simulink model "GazeboDifferentialDriveControl"  (R2023b)
settings: Solver=VariableStepAuto  StartTime=0.0  StopTime=15  RelTol=1e-3
StopFcn:
  | robotPoses = out.yout{1}.Values.Data;
  | 
  | figure;
  | plot(waypoints(:,1), waypoints(:,2), 'k-x');
  | hold all
  | plot(robotPoses(:,1), robotPoses(:,2));
  | title('XY Waypoint Tracking');
undefined symbols (not defined in the file): duration, effort, index, joint_name, left_wheel_hinge, model_name, pioneer2dx, right_wheel_hinge, waypoints
libraries: robotgazebolib x10, robotalgslib x1, robotcorelib x1
settings Model: PacingRate=0.011000  Creator=The MathWorks, Inc.  LastModifiedBy=basit
settings SolverCC: AlgebraicLoopSolver=TrustRegion
settings DebuggingCC: UnconnectedInputMsg=warning  UnconnectedOutputMsg=warning  UnconnectedLineMsg=warning  SymbolicDimsDataTypeCodeGenerationDiagnostic=none
settings ModelReferenceCC: EnableRefExpFcnMdlSchedulingChecks=on

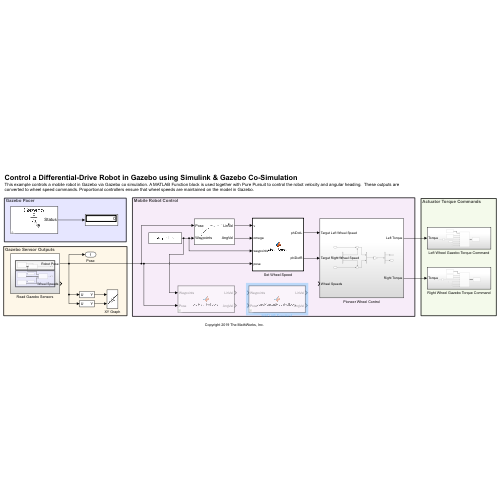
[thumbnail: Simulink's stored preview of the top-level diagram]
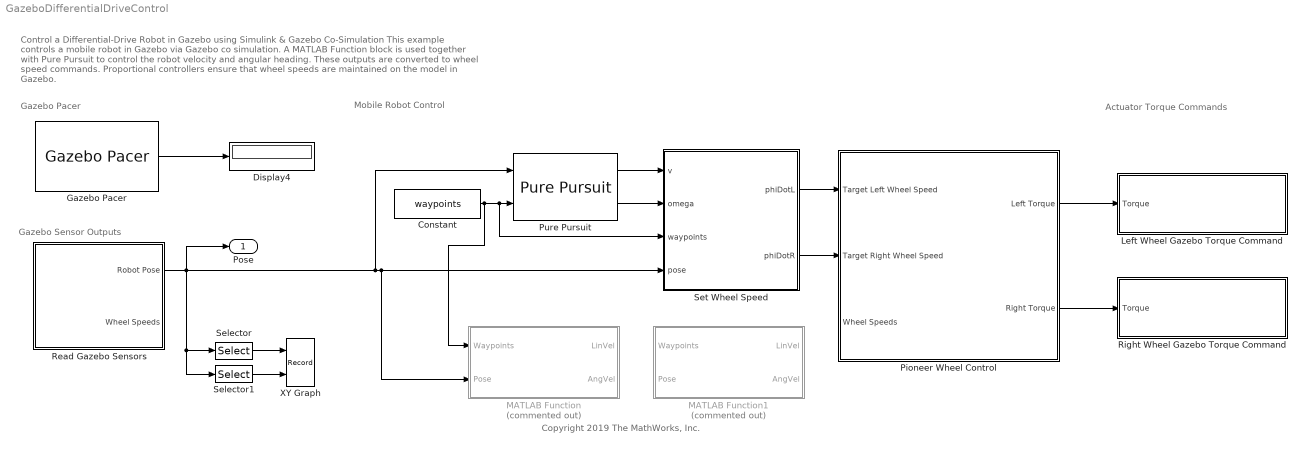
== system GazeboDifferentialDriveControl ==
  note: Gazebo Pacer
  note: Actuator Torque Commands
  note: Control a Differential-Drive Robot in Gazebo using Simulink & Gazebo Co-Simulation
      | This example controls a mobile robot in Gazebo via Gazebo co simulation. A MATLAB Function block is used together with Pure Pursuit to control the robot velocity and angular heading. These outputs are converted to wheel speed commands. Proportional controllers ensure that wheel speeds are maintained on the model in Gazebo.
  note: Copyright 2019 The MathWorks, Inc.
  note: Gazebo Sensor Outputs
  note: Mobile Robot Control
  Constant : Constant  Value=waypoints
  Display4 : Display
  Gazebo Pacer : robotgazebolib/Gazebo Pacer  ResetBehavior=Reset Gazebo simulation time and scene  SampleTime=0.01
  Left Wheel Gazebo Torque Command : Subsystem
  MATLAB Function : MATLAB Function  Commented=on  TreatAsAtomicUnit=on
  MATLAB Function1 : MATLAB Function  Commented=on  TreatAsAtomicUnit=on
  Pioneer Wheel Control : Subsystem
  Pure Pursuit : robotalgslib/Pure Pursuit  DesiredLinearVelocity=1  MaxAngularVelocity=1.0  LookaheadDistance=1.0  TargetDirPort=off  SimulateUsing=Code generation
  Read Gazebo Sensors : Subsystem
  Right Wheel Gazebo Torque Command : Subsystem
  Selector : Selector  InputPortWidth=3  IndexOptions=Index vector (dialog)  Indices=[1]  OutputSizes=1
  Selector1 : Selector  InputPortWidth=3  IndexOptions=Index vector (dialog)  Indices=[2]  OutputSizes=1
  Set Wheel Speed : MATLAB Function  TreatAsAtomicUnit=on
  XY Graph : Record  FileSettingsInternal="{\"entries\":[{\"content\":{\"excelSettings\":{\"content\":{},\"type\":\"Streamout.ExcelSettings\"}},\"type\":\"Streamout.FileSettingStorage\",\"uuid\":\"\"}],\"packageUris\":[\"http:\\/\\/schema.mathworks.com\\/mf0\\/streamout_blocks\\/R2020a\"],\"version\":\"1.0\"}"  Layout=[1 1]  SignalsInternal="{\"entries\":[{\"content\":{\"signals\":[{\"content\":{\"blockPath\":[],\"dimensions\":[1],\"domain\":\"\",\"lineColor\":\"#a2142f\",\"port\":1,\"signalID\":8,\"signalName\":\"XY Graph:1\"},\"type\":\"RecordBlkView.Signal\",\"uuid\":\"\"},{\"content\":{\"blockPath\":[],\"dimensions\":[1],\"domain\":\"\",\"lineColor\":\"#139fff\",\"plots\":[1],\"port\":2,\"signalID\":11,\"signalName\":\"XY Graph:2\"},\"type\":\"RecordBlkView.Signal\",\"uuid\":\"\"}]},\"type\":\"RecordBlkView.InputSignals\",\"uuid\":\"\"}],\"packageUris\":[\"http:\\/\\/schema.mathworks.com\\/mf0\\/streamout_blocks\\/R2020a\"],\"version\":\"1.0\"}"  VisualizationBindings="{\"xyplotplugin\":{\"info\":[{\"series\":[{\"bindingParametersList\":[{\"parameter\":\"Y-Axis\",\"signalID\":11,\"signalName\":\"XY Graph:2\"}],\"seriesID\":42836}],\"subplotID\":1}]}}"  CompatibilityTag=XY  st=-1
  Pose : Outport
  wires:
  Set Wheel Speed/1(phiDotL) -> Pioneer Wheel Control/1(Target Left Wheel Speed)
  Gazebo Pacer/1 -> Display4/1
  Constant/1 -> MATLAB Function/1(Waypoints), Set Wheel Speed/3(waypoints), Pure Pursuit/2
  Read Gazebo Sensors/1(Robot Pose) -> MATLAB Function/2(Pose), Set Wheel Speed/4(pose), Pure Pursuit/1, Pose/1, Selector/1, Selector1/1
  Pioneer Wheel Control/1(Left Torque) -> Left Wheel Gazebo Torque Command/1(Torque)
  Pioneer Wheel Control/2(Right Torque) -> Right Wheel Gazebo Torque Command/1(Torque)
  Selector/1 -> XY Graph/1
  Selector1/1 -> XY Graph/2
  Pure Pursuit/1 -> Set Wheel Speed/1(v)
  Pure Pursuit/2 -> Set Wheel Speed/2(omega)
  Set Wheel Speed/2(phiDotR) -> Pioneer Wheel Control/2(Target Right Wheel Speed)

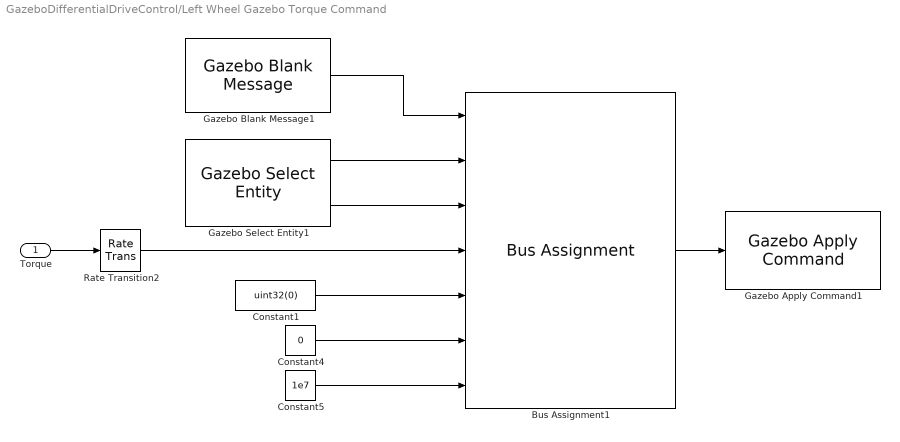
== system GazeboDifferentialDriveControl/Left Wheel Gazebo Torque Command ==
  Torque : Inport
  Bus Assignment1 : BusAssignment  AssignedSignals=model_name,joint_name,effort,index,duration.seconds,duration.nano_seconds
  Constant1 : Constant  Value=uint32(0)
  Constant4 : Constant  Value=0
  Constant5 : Constant  Value=1e7
  Gazebo Apply Command1 : robotgazebolib/Gazebo Apply Command  cmdType=ApplyJointTorque  sampleTime=0.01
  Gazebo Blank Message1 : robotgazebolib/Gazebo Blank Message  msgType=ApplyJointTorque  sampleTime=0.01  busName='Gazebo_SL_Bus_gazebo_msgs_ApplyJointTorque'
  Gazebo Select Entity1 : robotgazebolib/Gazebo Select Entity  modelElemName=pioneer2dx/left_wheel_hinge  outputArraySize=128  OutputLabel=Joint  SelectType=Joint
  Rate Transition2 : RateTransition
  wires:
  Bus Assignment1/1 -> Gazebo Apply Command1/1
  Constant5/1 -> Bus Assignment1/7
  Gazebo Blank Message1/1 -> Bus Assignment1/1
  Gazebo Select Entity1/2 -> Bus Assignment1/3
  Gazebo Select Entity1/1 -> Bus Assignment1/2
  Torque/1 -> Rate Transition2/1
  Constant4/1 -> Bus Assignment1/6
  Rate Transition2/1 -> Bus Assignment1/4
  Constant1/1 -> Bus Assignment1/5

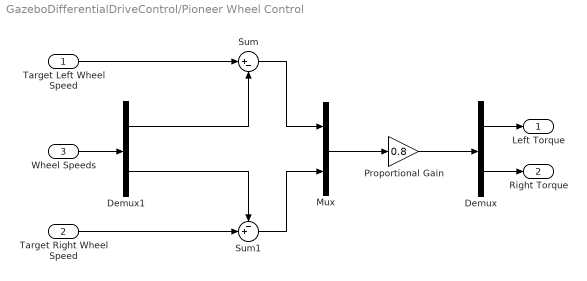
== system GazeboDifferentialDriveControl/Pioneer Wheel Control ==
  Target Left Wheel Speed : Inport
  Target Right Wheel Speed : Inport  Port=2
  Wheel Speeds : Inport  Port=3
  Demux : Demux  Outputs=2
  Demux1 : Demux  Outputs=2
  Mux : Mux  Inputs=2
  Proportional Gain : Gain  Gain=0.8
  Sum : Sum  Inputs=|+-
  Sum1 : Sum  Inputs=-+|
  Left Torque : Outport
  Right Torque : Outport  Port=2
  wires:
  Sum1/1 -> Mux/2
  Target Left Wheel Speed/1 -> Sum/1
  Sum/1 -> Mux/1
  Mux/1 -> Proportional Gain/1
  Proportional Gain/1 -> Demux/1
  Demux/1 -> Left Torque/1
  Demux/2 -> Right Torque/1
  Wheel Speeds/1 -> Demux1/1
  Demux1/1 -> Sum/2
  Target Right Wheel Speed/1 -> Sum1/2
  Demux1/2 -> Sum1/1

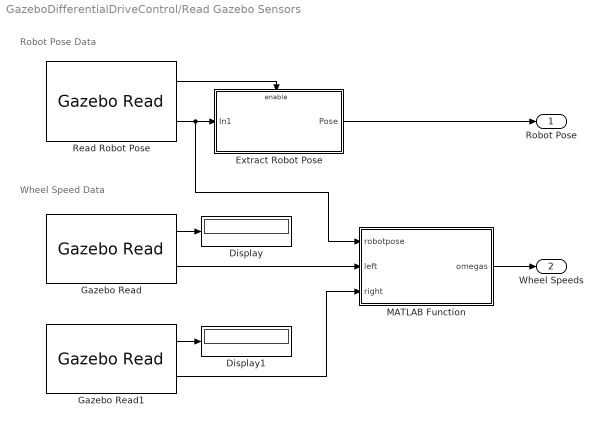
== system GazeboDifferentialDriveControl/Read Gazebo Sensors ==
  note: Robot Pose Data
  note: Wheel Speed Data
  Display : Display
  Display1 : Display
  Extract Robot Pose : Subsystem
  Gazebo Read : robotgazebolib/Gazebo Read  topicSource=From Gazebo  topic=/gazebo/ground_truth/world_pose/pioneer2dx/left_wheel  messageType=gazebo_msgs/Pose  sampleTime=0.01  fixedAxisBusStatus=off  jointAxisCount=2
  Gazebo Read1 : robotgazebolib/Gazebo Read  topicSource=From Gazebo  topic=/gazebo/ground_truth/world_pose/pioneer2dx/right_wheel  messageType=gazebo_msgs/Pose  sampleTime=0.01  fixedAxisBusStatus=off  jointAxisCount=2
  MATLAB Function : MATLAB Function  TreatAsAtomicUnit=on
  Read Robot Pose : robotgazebolib/Gazebo Read  topicSource=From Gazebo  topic=/gazebo/ground_truth/world_pose/pioneer2dx/chassis  messageType=gazebo_msgs/Pose  sampleTime=0.01  fixedAxisBusStatus=off  jointAxisCount=2
  Robot Pose : Outport
  Wheel Speeds : Outport  Port=2
  wires:
  Read Robot Pose/2 -> MATLAB Function/1(robotpose), Extract Robot Pose/1(In1)
  Extract Robot Pose/1(Pose) -> Robot Pose/1
  Read Robot Pose/1 -> Extract Robot Pose/Enable
  Gazebo Read/1 -> Display/1
  Gazebo Read1/1 -> Display1/1
  MATLAB Function/1(omegas) -> Wheel Speeds/1
  Gazebo Read/2 -> MATLAB Function/2(left)
  Gazebo Read1/2 -> MATLAB Function/3(right)

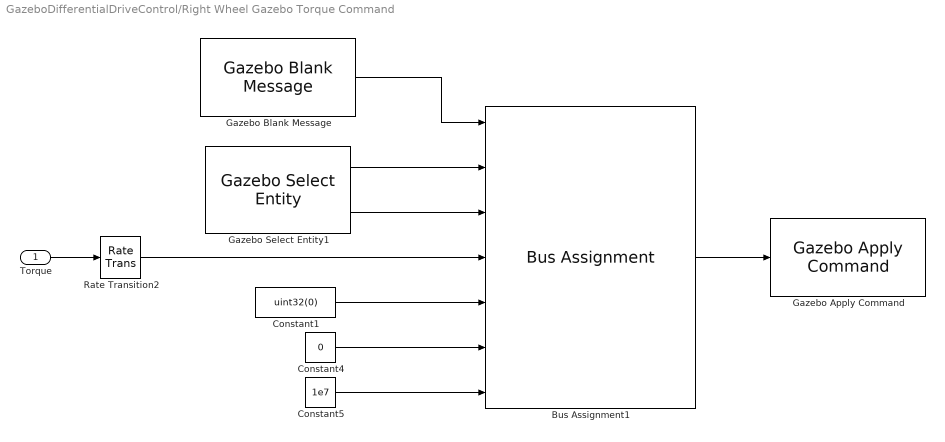
== system GazeboDifferentialDriveControl/Right Wheel Gazebo Torque Command ==
  Torque : Inport
  Bus Assignment1 : BusAssignment  AssignedSignals=model_name,joint_name,effort,index,duration.seconds,duration.nano_seconds
  Constant1 : Constant  Value=uint32(0)
  Constant4 : Constant  Value=0
  Constant5 : Constant  Value=1e7
  Gazebo Apply Command : robotgazebolib/Gazebo Apply Command  cmdType=ApplyJointTorque  sampleTime=0.01
  Gazebo Blank Message : robotgazebolib/Gazebo Blank Message  msgType=ApplyJointTorque  sampleTime=0.01  busName='Gazebo_SL_Bus_gazebo_msgs_ApplyJointTorque'
  Gazebo Select Entity1 : robotgazebolib/Gazebo Select Entity  modelElemName=pioneer2dx/right_wheel_hinge  outputArraySize=128  OutputLabel=Joint  SelectType=Joint
  Rate Transition2 : RateTransition
  wires:
  Constant1/1 -> Bus Assignment1/5
  Rate Transition2/1 -> Bus Assignment1/4
  Constant4/1 -> Bus Assignment1/6
  Torque/1 -> Rate Transition2/1
  Gazebo Select Entity1/1 -> Bus Assignment1/2
  Gazebo Select Entity1/2 -> Bus Assignment1/3
  Gazebo Blank Message/1 -> Bus Assignment1/1
  Constant5/1 -> Bus Assignment1/7
  Bus Assignment1/1 -> Gazebo Apply Command/1

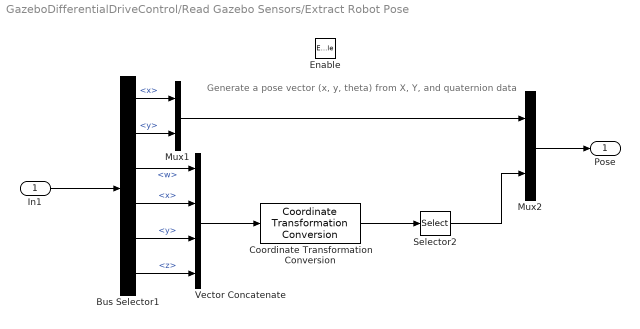
== system GazeboDifferentialDriveControl/Read Gazebo Sensors/Extract Robot Pose ==
  note: Generate a pose vector (x, y, theta) from X, Y, and quaternion data
  In1 : Inport
  Enable : EnablePort
  Bus Selector1 : BusSelector  OutputSignals=position.x,position.y,orientation.w,orientation.x,orientation.y,orientation.z
  Coordinate Transformation Conversion : robotcorelib/Coordinate Transformation Conversion  InputRepresentation=Quaternion  InputEulerSequence=ZYX  ShowTrVecInputPort=on  OutputRepresentation=Euler Angles  OutputEulerSequence=ZYX  ShowTrVecOutputPort=on  SimulateUsing=Interpreted execution
  Mux1 : Mux  Inputs=2
  Mux2 : Mux  Inputs=2
  Selector2 : Selector  InputPortWidth=3  IndexOptions=Index vector (dialog)  Indices=1  OutputSizes=1
  Vector Concatenate : Concatenate  NumInputs=4
  Pose : Outport  VectorParamsAs1DForOutWhenUnconnected=off
  wires:
  Vector Concatenate/1 -> Coordinate Transformation Conversion/1
  Coordinate Transformation Conversion/1 -> Selector2/1
  Mux1/1 -> Mux2/1
  Selector2/1 -> Mux2/2
  Mux2/1 -> Pose/1
  Bus Selector1/6 -> Vector Concatenate/4  "<z>"
  Bus Selector1/1 -> Mux1/1  "<x>"
  Bus Selector1/4 -> Vector Concatenate/2  "<x>"
  Bus Selector1/2 -> Mux1/2  "<y>"
  Bus Selector1/3 -> Vector Concatenate/1  "<w>"
  Bus Selector1/5 -> Vector Concatenate/3  "<y>"
  In1/1 -> Bus Selector1/1

== matlab function GazeboDifferentialDriveControl/Read Gazebo Sensors/MATLAB Function ==
  data: robotpose input; omegas output; left input; right input
function omegas = computeWheelVelocities(robotpose, left, right)
%computeWheelVelocities computes wheel velocity based on rate of change of
%the yaw angle of the wheel relative to its original mount on the robot
%body

persistent initAngles
if isempty(initAngles)
    initAngles = zeros(2,1);
end
sampleTime = 0.01;

% compute rotation between wheel original mount on the robot body and world
% frame
robotRtom = quat2rotm([robotpose.orientation.w, robotpose.orientation.x, robotpose.orientation.y, robotpose.orientation.z]);
originalWheelMount = robotRtom*eul2rotm([pi/2 pi/2 0]);

% get rotation between wheel and the world frame
leftRtom = quat2rotm([left.orientation.w, left.orientation.x, left.orientation.y, left.orientation.z]);
rightRtom = quat2rotm([right.orientation.w, right.orientation.x, right.orientation.y, right.orientation.z]);

% compute relative rotation between wheel and its original mount
leftRotation = rotm2eul(originalWheelMount'*leftRtom);
rightRotation = rotm2eul(originalWheelMount'*rightRtom);

% compute angluar velocity using the angle difference between the current
% angle pose and the the angle pose in last time step
angles = [leftRotation(1); rightRotation(1)];
omegas = angdiff(initAngles, angles)/sampleTime;
initAngles = angles;

== matlab function GazeboDifferentialDriveControl/Set Wheel Speed ==
  data: v input; omega input; waypoints input; pose input; phiDotL output; phiDotR output
function [phiDotL, phiDotR] = wheelSpeed(v, omega, waypoints, pose)

% Path constants
stopThreshold = 0.1;
slowThreshold = 0.3;

% Robot constants
trackWidth = 0.381;
wheelRadius = 0.195/2;

% Slow the robot down when it's near the threshold
distanceToEndpoint = norm(waypoints(end, :) - pose(1:2)');
if (distanceToEndpoint < slowThreshold)
    v = distanceToEndpoint/slowThreshold*v;
    
    % Stop the robot if it's inside the target threshold
    if distanceToEndpoint < stopThreshold
        v = 0;
    end
end

% Convert velocity and heading angular velocity to wheel speeds
phiDotL = (v - trackWidth/2*omega)/wheelRadius;
phiDotR = (v + trackWidth/2*omega)/wheelRadius;

end

== matlab function GazeboDifferentialDriveControl/MATLAB Function ==
  data: Waypoints input; LinVel output; AngVel output; Pose input
function [LinVel, AngVel] = pidPathFollower(Waypoints,Pose)

== matlab function GazeboDifferentialDriveControl/MATLAB Function1 ==
  data: Waypoints input; LinVel output; AngVel output; Pose input
function [LinVel, AngVel] = purePursuitPathFollower(Waypoints,Pose)
